simulink model "Rocket_trajectory"  (R2018a)
settings: Solver=ode45  StartTime=0.0  StopTime=360  MinStep=1e-6  RelTol=1e-7
undefined symbols (not defined in the file): Ae, Azimuth, BurnoutInertia, BurnTime, CA, CG, CLL, CLLp, CLNb, CLNr, CMa, CMadot, CMq, CNa, CYb, deg, Earth, Finalcg, Fuel_mass, InertiaRate, InitialInertia, Initialmass, Lat, Launch_angle, Launch_site, Lon, Lref, MACH, Mass_flow, omegajeta, omegalox, rad, Ramup_time, s, Sample_time, Thrust, Thrust_time, Time_cg, Time_slosh, WGS84, Xref
libraries: aerolibconvert2 x6, simulink_extras x5, aerolibbdyn x4, aerolibwind2 x3, aerolibasang x3, aerolibtransform2 x2, aerolibatmos2 x1, shared6dof x1, aerolibfltsims x1, aerolibadyn x1
settings Model: Creator=mario  LastModifiedBy=mario
settings SolverCC: InitialStep=1e-6
settings CodeAppCC: StateflowObjectComments=on

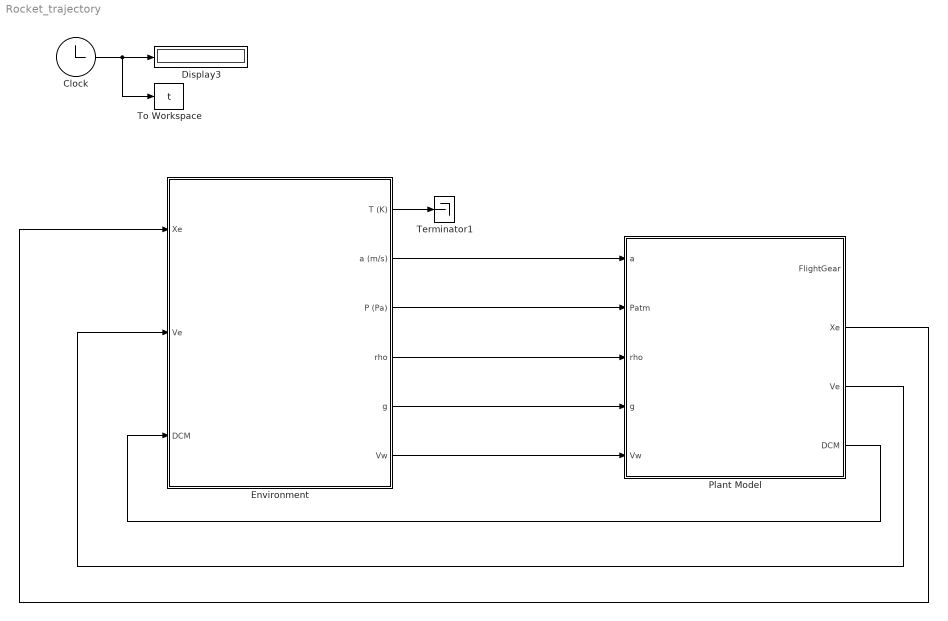
== system Rocket_trajectory ==
  Clock : Clock
  Display3 : Display
  Environment : Subsystem
  Plant Model : Subsystem
  Terminator1 : Terminator
  To Workspace : ToWorkspace  VariableName=t  SampleTime=Sample_time
  wires:
  Environment/3(P (Pa)) -> Plant Model/2(Patm)
  Environment/2(a (m/s)) -> Plant Model/1(a)
  Environment/6(Vw) -> Plant Model/5(Vw)
  Environment/5(g) -> Plant Model/4(g)
  Environment/1(T (K)) -> Terminator1/1
  Clock/1 -> To Workspace/1, Display3/1
  Plant Model/2(Xe) -> Environment/1(Xe)
  Environment/4("rho ") -> Plant Model/3(rho)
  Plant Model/4(DCM) -> Environment/3(DCM)
  Plant Model/3(Ve) -> Environment/2(Ve)

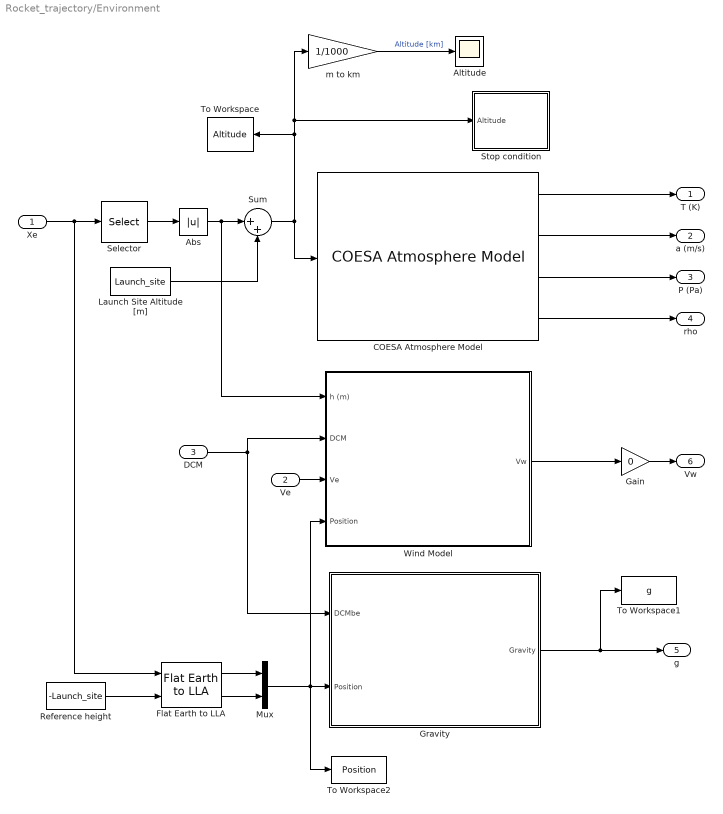
== system Rocket_trajectory/Environment ==
  Xe : Inport
  Ve : Inport  Port=2
  DCM : Inport  Port=3
  Abs : Abs
  Altitude : Scope
  COESA Atmosphere Model : aerolibatmos2/COESA Atmosphere Model  units=Metric (MKS)  spec=1976 COESA-extended U.S. Standard Atmosphere  model=Profile  profile_var=High temperature  profile_percent=1%  profile_alt=5 km (16404 ft)  envelope_var=High temperature  envelope_percent=1%  action=Warning
  Flat Earth to LLA : aerolibtransform2/Flat Earth to LLA  units=Metric (MKS)  ptype=Earth (WGS84)  F=1/298.257223563  R=6378137  LL0=[Lat Lon]  psi=Azimuth
  Gain : Gain  Gain=0
  Gravity : Subsystem
  Launch Site Altitude [m] : Constant  Value=Launch_site
  Mux : Mux  Inputs=2
  Reference height : Constant  Value=-Launch_site
  Selector : Selector  InputPortWidth=3  IndexOptions=Index vector (dialog)  Indices=[3]  OutputSizes=1
  Stop condition : Subsystem
  Sum : Sum  Inputs=|++
  To Workspace : ToWorkspace  VariableName=Altitude  SampleTime=Sample_time
  To Workspace1 : ToWorkspace  VariableName=g  SampleTime=Sample_time
  To Workspace2 : ToWorkspace  VariableName=Position  SampleTime=Sample_time
  Wind Model : Subsystem
  m to km : Gain  Gain=1/1000
  T (K) : Outport
  a (m/s) : Outport  Port=2
  P (Pa) : Outport  Port=3
  "rho " : Outport  Port=4
  g : Outport  Port=5
  Vw : Outport  Port=6
  wires:
  Launch Site Altitude [m]/1 -> Sum/2
  m to km/1 -> Altitude/1  "Altitude [km]"
  Selector/1 -> Abs/1
  COESA Atmosphere Model/2 -> a (m/s)/1
  COESA Atmosphere Model/1 -> T (K)/1
  Abs/1 -> Wind Model/1(h (m)), Sum/1
  Xe/1 -> Selector/1, Flat Earth to LLA/1
  COESA Atmosphere Model/3 -> P (Pa)/1
  COESA Atmosphere Model/4 -> "rho "/1
  Sum/1 -> COESA Atmosphere Model/1, Stop condition/1(Altitude), m to km/1, To Workspace/1
  Ve/1 -> Wind Model/3(Ve)
  Gravity/1(Gravity) -> To Workspace1/1, g/1
  DCM/1 -> Wind Model/2(DCM), Gravity/1(DCMbe)
  Flat Earth to LLA/1 -> Mux/1
  Flat Earth to LLA/2 -> Mux/2
  Mux/1 -> To Workspace2/1, Wind Model/4(Position), Gravity/2(Position)
  Reference height/1 -> Flat Earth to LLA/2
  Gain/1 -> Vw/1
  Wind Model/1(Vw) -> Gain/1

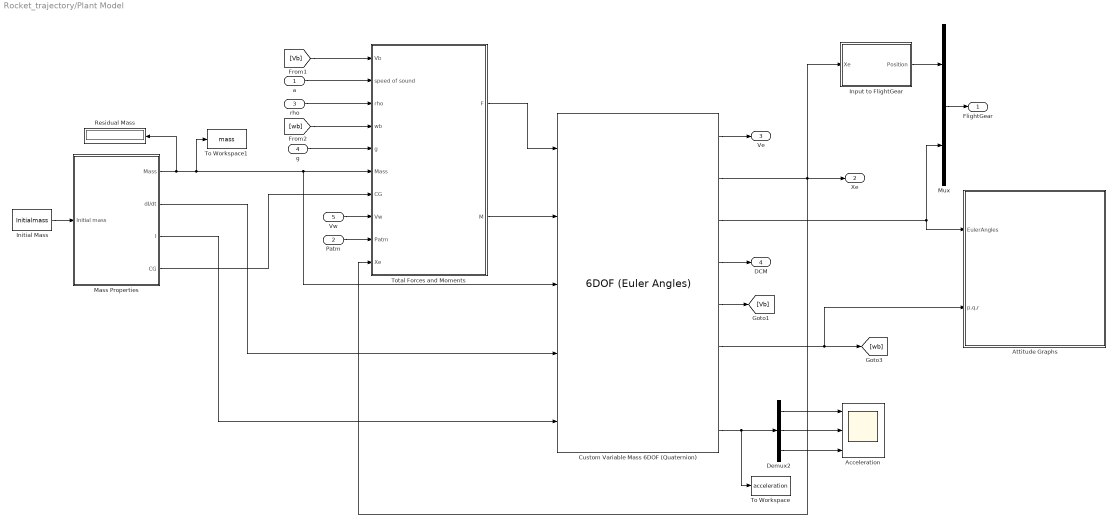
== system Rocket_trajectory/Plant Model ==
  a : Inport
  Patm : Inport  Port=2
  rho : Inport  Port=3
  g : Inport  Port=4
  Vw : Inport  Port=5
  Acceleration : Scope  NumInputPorts=3
  Attitude Graphs : Subsystem
  Custom Variable Mass 6DOF (Quaternion) : shared6dof/6DOF (Euler Angles)  units=Metric (MKS)  mtype=Custom Variable  rep=Quaternion  xme_0=[0 0 0]  Vm_0=[0.1 0.1 0.1]  eul_0=[0 Launch_angle Azimuth]  pm_0=[0 0 0]  mass_0=1.0  mass_e=0.5  mass_f=2.0  inertia=eye(3)  inertia_e=eye(3)  inertia_f=2*eye(3)  k_quat=1.0  vre_flag=off  abi_flag=off  aMode=aMode
      settings: SourceProductBaseCode=AE
  Demux2 : Demux  Outputs=3
  Initial Mass : Constant  Value=Initialmass
  Input to FlightGear : Subsystem
  Mass Properties : Subsystem
  Mux : Mux  Inputs=2
  Residual Mass : Display
  To Workspace : ToWorkspace  VariableName=acceleration  SampleTime=Sample_time
  To Workspace1 : ToWorkspace  VariableName=mass  SampleTime=Sample_time
  "Total Forces and Moments " : Subsystem
  FlightGear : Outport
  Xe : Outport  Port=2
  Ve : Outport  Port=3
  DCM : Outport  Port=4
  wires:
  Custom Variable Mass 6DOF (Quaternion)/4 -> DCM/1
  Mux/1 -> FlightGear/1
  Custom Variable Mass 6DOF (Quaternion)/6 -> [wb], Attitude Graphs/2(p,q,r)
  Custom Variable Mass 6DOF (Quaternion)/1 -> Ve/1
  "Total Forces and Moments "/2("M ") -> Custom Variable Mass 6DOF (Quaternion)/2
  Custom Variable Mass 6DOF (Quaternion)/3 -> Attitude Graphs/1(EulerAngles), Mux/2
  Custom Variable Mass 6DOF (Quaternion)/5 -> [Vb]
  [Vb] -> "Total Forces and Moments "/1("Vb ")
  Input to FlightGear/1(Position) -> Mux/1
  g/1 -> "Total Forces and Moments "/5(g)
  Demux2/3 -> Acceleration/3
  "Total Forces and Moments "/1(F) -> Custom Variable Mass 6DOF (Quaternion)/1
  Custom Variable Mass 6DOF (Quaternion)/2 -> "Total Forces and Moments "/10(Xe), Xe/1, Input to FlightGear/1(Xe)
  [wb] -> "Total Forces and Moments "/4(wb)
  Demux2/2 -> Acceleration/2
  rho/1 -> "Total Forces and Moments "/3("rho ")
  Demux2/1 -> Acceleration/1
  Custom Variable Mass 6DOF (Quaternion)/8 -> To Workspace/1, Demux2/1
  a/1 -> "Total Forces and Moments "/2(speed of sound)
  Mass Properties/2(dI/dt) -> Custom Variable Mass 6DOF (Quaternion)/4
  Initial Mass/1 -> Mass Properties/1(Initial mass)
  Mass Properties/1(Mass) -> To Workspace1/1, Custom Variable Mass 6DOF (Quaternion)/3, "Total Forces and Moments "/6(Mass), Residual Mass/1
  Mass Properties/3(I) -> Custom Variable Mass 6DOF (Quaternion)/5
  Mass Properties/4(CG) -> "Total Forces and Moments "/7(CG)
  Vw/1 -> "Total Forces and Moments "/8(Vw)
  Patm/1 -> "Total Forces and Moments "/9(Patm)

== system Rocket_trajectory/Environment/Gravity ==
  DCMbe : Inport
  Position : Inport  Port=2
  Display4 : Display
  Display5 : Display
  Product3 : Product  Multiplication=Matrix(*)
  "WGS84 Gravity Model  " : GravityWGS84
  Gravity : Outport
  wires:
  Product3/1 -> Gravity/1, Display4/1
  "WGS84 Gravity Model  "/1 -> Product3/2, Display5/1
  DCMbe/1 -> Product3/1
  Position/1 -> "WGS84 Gravity Model  "/1

== system Rocket_trajectory/Environment/Stop condition ==
  Altitude : Inport
  Clock : Clock
  Constant : Constant  Value=0
  Constant1 : Constant
  Constant2 : Constant  Value=Launch_site+10
  Stop Simulation : Stop
  Switch : Switch  Criteria=u2 > Threshold  Threshold=Launch_site+1
  Switch1 : Switch  Criteria=u2 > Threshold  Threshold=10
  wires:
  Switch/1 -> Stop Simulation/1
  Constant/1 -> Switch/1
  Constant1/1 -> Switch/3
  Altitude/1 -> Switch1/1
  Switch1/1 -> Switch/2
  Clock/1 -> Switch1/2
  Constant2/1 -> Switch1/3

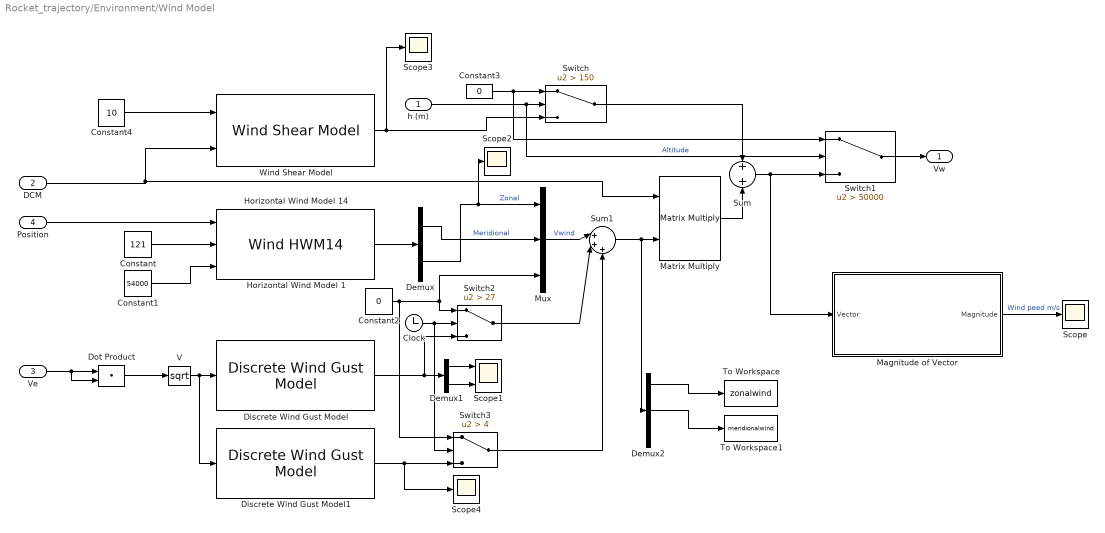
== system Rocket_trajectory/Environment/Wind Model ==
  h (m) : Inport
  DCM : Inport  Port=2
  Ve : Inport  Port=3
  Position : Inport  Port=4
  Clock : Clock
  Constant : Constant  Value=121
  Constant1 : Constant  Value=54000
  Constant2 : Constant  Value=0
  Constant3 : Constant  Value=0
  Constant4 : Constant  Value=10
  Demux : Demux  Outputs=2
  Demux1 : Demux  Outputs=2
  Demux2 : Demux  Outputs=3
  Discrete Wind Gust Model : aerolibwind2/Discrete Wind Gust Model  units=Metric (MKS)  Gx=on  Gy=on  Gz=off  t_0=20  d_m=[150 150 50]  v_m=[10 0 0]
      settings: SourceProductName=Aerospace Blockset
  Discrete Wind Gust Model1 : aerolibwind2/Discrete Wind Gust Model  units=Metric (MKS)  Gx=on  Gy=on  Gz=off  t_0=1  d_m=[20 20 8]  v_m=[10 0 0]
      settings: SourceProductName=Aerospace Blockset
  Dot Product : DotProduct  SaturateOnIntegerOverflow=on  OutDataTypeStr=Inherit: Inherit via internal rule
  Horizontal Wind Model 1 : WindHWM14
  Horizontal Wind Model 14 : WindHWM14
  Magnitude of Vector : Subsystem
  Matrix Multiply : Product  Multiplication=Matrix(*)
  Mux : Mux  Inputs=3
  Scope{,2..4} (4 alike) : Scope
  Scope1 : Scope  NumInputPorts=2
  Sum : Sum
  Sum1 : Sum  Inputs=|+++
  Switch : Switch  Criteria=u2 > Threshold  Threshold=150
  Switch1 : Switch  Criteria=u2 > Threshold  Threshold=50000
  Switch2 : Switch  Criteria=u2 > Threshold  Threshold=27
  Switch3 : Switch  Criteria=u2 > Threshold  Threshold=4
  To Workspace : ToWorkspace  VariableName=zonalwind  SampleTime=Sample_time
  To Workspace1 : ToWorkspace  VariableName=meridionalwind  SampleTime=Sample_time
  V : Math  Operator=sqrt  SaturateOnIntegerOverflow=on
  Wind Shear Model : aerolibwind2/Wind Shear Model  units=Metric (MKS)  phase=Category C - Terminal Flight Phase  W_20=10  Wdeg=20
      settings: SourceProductName=Aerospace Blockset
  Vw : Outport
  wires:
  Ve/1 -> Dot Product/2, Dot Product/1
  Dot Product/1 -> V/1
  Magnitude of Vector/1(Magnitude) -> Scope/1  "Wind peed m/s"
  Discrete Wind Gust Model/1 -> Switch2/3, Demux1/1
  Position/1 -> Horizontal Wind Model 14/1
  Constant/1 -> Horizontal Wind Model 14/2
  Constant1/1 -> Horizontal Wind Model 14/3
  Horizontal Wind Model 14/1 -> Demux/1
  Demux/1 -> Mux/2  "Meridional"
  Demux/2 -> Scope2/1, Mux/1  "Zonal"
  Demux1/1 -> Scope1/1
  Demux1/2 -> Scope1/2
  DCM/1 -> Wind Shear Model/2, Matrix Multiply/1
  Mux/1 -> Sum1/1  "Vwind"
  Matrix Multiply/1 -> Sum/2
  h (m)/1 -> Switch1/2, Switch/2  "Altitude"
  Sum/1 -> Switch1/3, Magnitude of Vector/1(Vector)
  Wind Shear Model/1 -> Scope3/1, Switch/3
  Switch/1 -> Sum/1
  Constant3/1 -> Switch1/1, Switch/1
  Constant4/1 -> Wind Shear Model/1
  Switch1/1 -> Vw/1
  Sum1/1 -> Demux2/1, Matrix Multiply/2
  Switch2/1 -> Sum1/2
  Demux2/1 -> To Workspace/1
  Demux2/2 -> To Workspace1/1
  V/1 -> Discrete Wind Gust Model1/1, Discrete Wind Gust Model/1
  Discrete Wind Gust Model1/1 -> Scope4/1, Switch3/3
  Clock/1 -> Switch3/2, Switch2/2
  Constant2/1 -> Switch3/1, Mux/3, Switch2/1
  Switch3/1 -> Sum1/3

== system Rocket_trajectory/Plant Model/Attitude Graphs ==
  EulerAngles : Inport
  p,q,r : Inport  Port=2
  Angular Rates : Scope  NumInputPorts=3
  Atittude : Scope  NumInputPorts=6
  Demux : Demux  Outputs=3
  Demux1 : Demux  Outputs=3
  Euler Angles : Scope  NumInputPorts=3
  "Roll, Pitch, Yaw" : simulink_extras/Transformations/Radians to Degrees
  wires:
  Demux/1 -> Atittude/1, Euler Angles/1  "Roll"
  "Roll, Pitch, Yaw"/1 -> Demux/1
  Demux1/3 -> Angular Rates/3, Atittude/6  "Yaw rate"
  Demux1/2 -> Angular Rates/2, Atittude/5  "Pitch rate"
  Demux/3 -> Atittude/3, Euler Angles/3  "Yaw"
  Demux/2 -> Atittude/2, Euler Angles/2  "Pitch"
  Demux1/1 -> Angular Rates/1, Atittude/4  "Roll rate"
  EulerAngles/1 -> "Roll, Pitch, Yaw"/1
  p,q,r/1 -> Demux1/1

== system Rocket_trajectory/Plant Model/Input to FlightGear ==
  Xe : Inport
  Constant2 : Constant  Value=-Launch_site
  Demux2 : Demux  Outputs=2
  Demux3 : Demux  Outputs=3
  Flat Earth to LLA : aerolibtransform2/Flat Earth to LLA  units=Metric (MKS)  ptype=Earth (WGS84)  F=1/298.257223563  R=6378137  LL0=[Lat Lon]  psi=0
  Generate Run Script : aerolibfltsims/Generate Run Script  Architecture=Win64  dataFlow=Send  GeometryModelName=sr71  AirportId=KSFO  RunwayId=10L  InitialAltitude=4593  InitialHeading=0  OffsetDistance=4.72  OffsetAzimuth=0  InstallScenery=off  DisableShaders=off  OriginAddress=127.0.0.1  DestinationPort=5502  OriginPort=5505  LocalAddress=127.0.0.1  OutputFileName=runfg.bat  FlightGearBaseDirectory=C:\Program Files\FlightGear 2017.3.1
  Mux1 : Mux  Inputs=3
  Mux2 : Mux  Inputs=3
  Position : Outport
  wires:
  Demux3/3 -> Mux1/3
  Demux3/1 -> Mux1/1
  Flat Earth to LLA/2 -> Mux2/3
  Xe/1 -> Demux3/1
  Demux2/1 -> Mux2/2
  Demux2/2 -> Mux2/1
  Flat Earth to LLA/1 -> Demux2/1
  Constant2/1 -> Flat Earth to LLA/2
  Mux1/1 -> Flat Earth to LLA/1
  Demux3/2 -> Mux1/2
  Mux2/1 -> Position/1

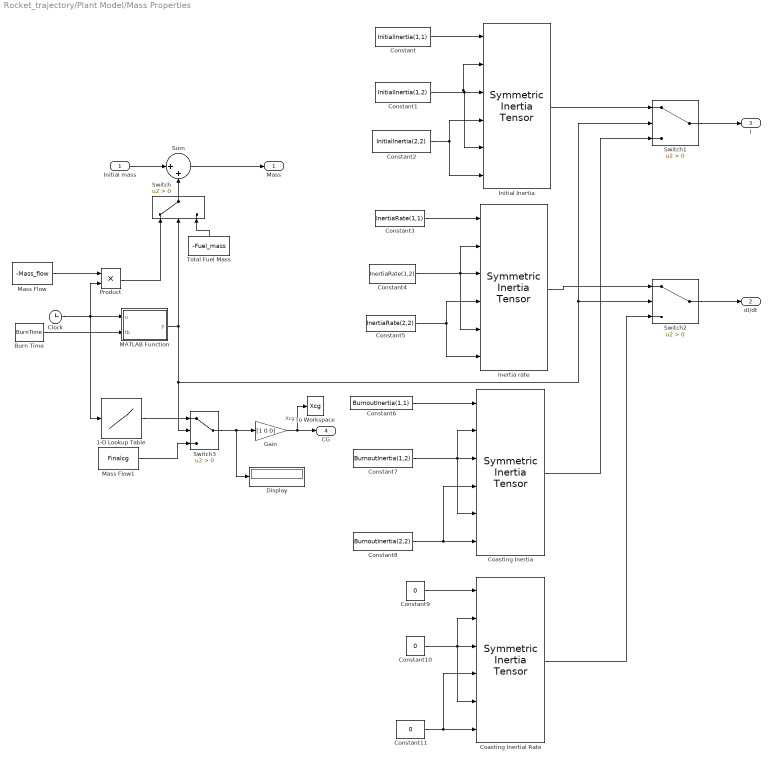
== system Rocket_trajectory/Plant Model/Mass Properties ==
  Initial mass : Inport
  1-D Lookup Table : Lookup_n-D  NumberOfTableDimensions=1  BreakpointsForDimension1=Time_cg  Table=CG  InternalRulePriority=Speed  RndMeth=Simplest  InputSameDT=on
  Burn Time : Constant  Value=BurnTime
  Clock : Clock
  Coasting Inertia : aerolibbdyn/Symmetric Inertia Tensor
      settings: SourceProductName=Aerospace Blockset  SourceProductBaseCode=AE
  Coasting Inertial Rate : aerolibbdyn/Symmetric Inertia Tensor
      settings: SourceProductName=Aerospace Blockset  SourceProductBaseCode=AE
  Constant : Constant  Value=InitialInertia(1,1)
  Constant1 : Constant  Value=InitialInertia(1,2)
  Constant10 : Constant  Value=0
  Constant11 : Constant  Value=0
  Constant2 : Constant  Value=InitialInertia(2,2)
  Constant3 : Constant  Value=InertiaRate(1,1)
  Constant4 : Constant  Value=InertiaRate(1,2)
  Constant5 : Constant  Value=InertiaRate(2,2)
  Constant6 : Constant  Value=BurnoutInertia(1,1)
  Constant7 : Constant  Value=BurnoutInertia(1,2)
  Constant8 : Constant  Value=BurnoutInertia(2,2)
  Constant9 : Constant  Value=0
  Display : Display
  Gain : Gain  Gain=[1 0 0]
  Inertia rate : aerolibbdyn/Symmetric Inertia Tensor
      settings: SourceProductName=Aerospace Blockset  SourceProductBaseCode=AE
  Initial Inertia : aerolibbdyn/Symmetric Inertia Tensor
      settings: SourceProductName=Aerospace Blockset  SourceProductBaseCode=AE
  MATLAB Function : MATLAB Function  TreatAsAtomicUnit=on
  Mass Flow : Constant  Value=-Mass_flow
  Mass Flow1 : Constant  Value=Finalcg
  Product : Product
  Sum : Sum  Inputs=|++
  Switch{,1..3} (4 alike) : Switch  Criteria=u2 > Threshold
  To Workspace : ToWorkspace  VariableName=Xcg  SampleTime=Sample_time
  Total Fuel Mass : Constant  Value=-Fuel_mass
  Mass : Outport
  dI/dt : Outport  Port=2
  I : Outport  Port=3
  CG : Outport  Port=4
  wires:
  Initial mass/1 -> Sum/1
  Constant/1 -> Initial Inertia/1
  Constant1/1 -> Initial Inertia/5, Initial Inertia/2, Initial Inertia/3
  Constant2/1 -> Initial Inertia/4, Initial Inertia/6
  Mass Flow/1 -> Product/1
  Clock/1 -> 1-D Lookup Table/1, Product/2, MATLAB Function/1(u)
  Product/1 -> Switch/1
  Constant5/1 -> Inertia rate/4, Inertia rate/6
  Constant3/1 -> Inertia rate/1
  Constant4/1 -> Inertia rate/2, Inertia rate/5, Inertia rate/3
  Inertia rate/1 -> Switch2/1
  Sum/1 -> Mass/1
  Switch/1 -> Sum/2
  Total Fuel Mass/1 -> Switch/3
  Burn Time/1 -> MATLAB Function/2(tb)
  Coasting Inertia/1 -> Switch1/3
  Constant8/1 -> Coasting Inertia/4, Coasting Inertia/6
  Constant6/1 -> Coasting Inertia/1
  Constant7/1 -> Coasting Inertia/5, Coasting Inertia/2, Coasting Inertia/3
  Initial Inertia/1 -> Switch1/1
  Switch1/1 -> I/1
  Switch2/1 -> dI/dt/1
  Constant11/1 -> Coasting Inertial Rate/4, Coasting Inertial Rate/6
  Constant9/1 -> Coasting Inertial Rate/1
  Constant10/1 -> Coasting Inertial Rate/2, Coasting Inertial Rate/3, Coasting Inertial Rate/5
  Coasting Inertial Rate/1 -> Switch2/3
  1-D Lookup Table/1 -> Switch3/1
  Switch3/1 -> Gain/1, Display/1
  MATLAB Function/1(y) -> Switch3/2, Switch2/2, Switch1/2, Switch/2
  Mass Flow1/1 -> Switch3/3
  Gain/1 -> To Workspace/1, CG/1  "Xcg"

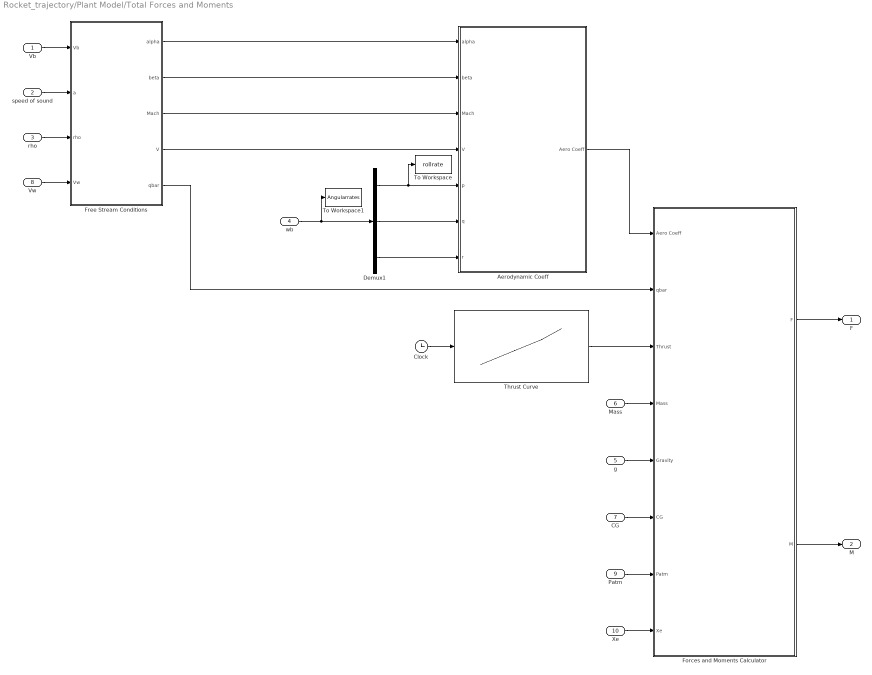
== system Rocket_trajectory/Plant Model/Total Forces and Moments  ==
  "Vb " : Inport
  speed of sound : Inport  Port=2
  "rho " : Inport  Port=3
  wb : Inport  Port=4
  g : Inport  Port=5
  Mass : Inport  Port=6
  CG : Inport  Port=7
  Vw : Inport  Port=8
  Patm : Inport  Port=9
  Xe : Inport  Port=10
  Aerodynamic Coeff : Subsystem
  Clock : Clock
  Demux1 : Demux  Outputs=3
  Forces and Moments Calculator : Subsystem
  Free Stream Conditions : Subsystem
  "Thrust Curve " : Lookup_n-D  NumberOfTableDimensions=1  BreakpointsForDimension1=Thrust_time  Table=Thrust  InternalRulePriority=Speed  RndMeth=Simplest  InputSameDT=on
  To Workspace : ToWorkspace  VariableName=rollrate  SampleTime=Sample_time
  To Workspace1 : ToWorkspace  VariableName=Angularrates  SampleTime=-1
  F : Outport
  "M " : Outport  Port=2
  wires:
  Aerodynamic Coeff/1(Aero Coeff) -> Forces and Moments Calculator/1(Aero Coeff)
  Forces and Moments Calculator/1(F) -> F/1
  Forces and Moments Calculator/2(M) -> "M "/1
  Mass/1 -> Forces and Moments Calculator/4(Mass)
  "Thrust Curve "/1 -> Forces and Moments Calculator/3(Thrust)
  Clock/1 -> "Thrust Curve "/1
  Demux1/3 -> Aerodynamic Coeff/7(r)
  Demux1/2 -> Aerodynamic Coeff/6(q)
  wb/1 -> To Workspace1/1, Demux1/1
  Demux1/1 -> To Workspace/1, Aerodynamic Coeff/5(p)
  g/1 -> Forces and Moments Calculator/5(Gravity)
  "Vb "/1 -> Free Stream Conditions/1(Vb)
  speed of sound/1 -> Free Stream Conditions/2(a)
  "rho "/1 -> Free Stream Conditions/3(rho)
  Free Stream Conditions/1(alpha) -> Aerodynamic Coeff/1(alpha)
  Free Stream Conditions/2(beta) -> Aerodynamic Coeff/2(beta)
  Free Stream Conditions/3(Mach) -> Aerodynamic Coeff/3(Mach)
  Free Stream Conditions/4(V) -> Aerodynamic Coeff/4(V)
  Free Stream Conditions/5(qbar) -> Forces and Moments Calculator/2(qbar)
  CG/1 -> Forces and Moments Calculator/6(CG)
  Vw/1 -> Free Stream Conditions/4(Vw)
  Patm/1 -> Forces and Moments Calculator/7(Patm)
  Xe/1 -> Forces and Moments Calculator/8(Xe)

== system Rocket_trajectory/Environment/Wind Model/Magnitude of Vector ==
  Vector : Inport
  Demux : Demux  Outputs=3
  Multiply : Product
  Multiply1 : Product
  Multiply2 : Product
  Sqrt : Sqrt  SaturateOnIntegerOverflow=on
  Sum1 : Sum  Inputs=3
  Magnitude : Outport
  wires:
  Demux/1 -> Multiply/2, Multiply/1
  Sum1/1 -> Sqrt/1
  Demux/2 -> Multiply1/1, Multiply1/2
  Multiply1/1 -> Sum1/2
  Sqrt/1 -> Magnitude/1
  Demux/3 -> Multiply2/2, Multiply2/1
  Multiply2/1 -> Sum1/3
  Multiply/1 -> Sum1/1
  Vector/1 -> Demux/1

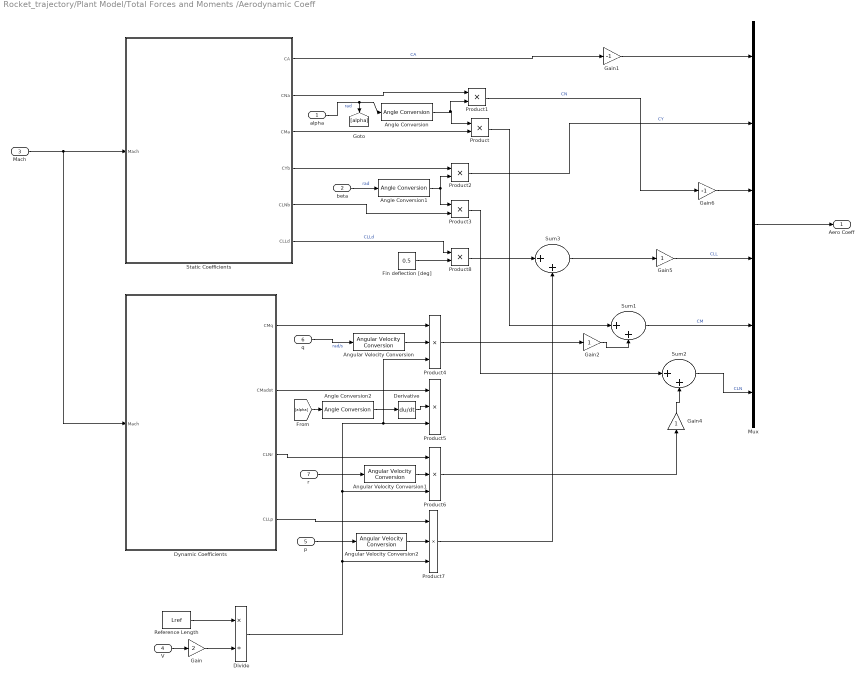
== system Rocket_trajectory/Plant Model/Total Forces and Moments /Aerodynamic Coeff ==
  alpha : Inport
  beta : Inport  Port=2
  Mach : Inport  Port=3
  V : Inport  Port=4
  p : Inport  Port=5
  q : Inport  Port=6
  r : Inport  Port=7
  Angle Conversion : aerolibconvert2/Angle Conversion  IU=rad  OU=deg
  Angle Conversion1 : aerolibconvert2/Angle Conversion  IU=rad  OU=deg
  Angle Conversion2 : aerolibconvert2/Angle Conversion  IU=rad  OU=deg
  Angular Velocity Conversion : aerolibconvert2/Angular Velocity Conversion  IU=rad/s  OU=deg/s
      settings: SourceProductName=Aerospace Blockset
  Angular Velocity Conversion1 : aerolibconvert2/Angular Velocity Conversion  IU=rad/s  OU=deg/s
      settings: SourceProductName=Aerospace Blockset
  Angular Velocity Conversion2 : aerolibconvert2/Angular Velocity Conversion  IU=rad/s  OU=deg/s
      settings: SourceProductName=Aerospace Blockset
  Derivative : Derivative
  Divide : Product  Inputs=*/
  Dynamic Coefficients : Subsystem
  Fin deflection [deg] : Constant  Value=0.5
  Gain : Gain  Gain=2
  Gain1 : Gain  Gain=-1
  Gain2 : Gain
  Gain4 : Gain
  Gain5 : Gain
  Gain6 : Gain  Gain=-1
  Mux : Mux  Inputs=6
  Product{,1..3,8} (5 alike) : Product
  Product{4..7} (4 alike) : Product  Inputs=3
  Reference Length : Constant  Value=Lref
  "Static Coefficients " : Subsystem
  Sum1 : Sum  Inputs=|++
  Sum2 : Sum  Inputs=|++
  Sum3 : Sum  Inputs=|++
  Aero Coeff : Outport
  wires:
  Mach/1 -> "Static Coefficients "/1(Mach), Dynamic Coefficients/1(Mach)
  Dynamic Coefficients/1("CMq ") -> Product4/1
  Mux/1 -> Aero Coeff/1
  "Static Coefficients "/1("CA ") -> Gain1/1  "CA"
  Product1/1 -> Gain6/1  "CN"
  "Static Coefficients "/6("CLLd  ") -> Product8/1  "CLLd"
  Sum1/1 -> Mux/5  "CM"
  Sum2/1 -> Mux/6  "CLN"
  alpha/1 -> Angle Conversion/1, [alpha]  "rad"
  "Static Coefficients "/3("CMa ") -> Product/2
  "Static Coefficients "/2("CNa ") -> Product1/1
  beta/1 -> Angle Conversion1/1  "rad"
  "Static Coefficients "/5("CLNb ") -> Product3/2
  "Static Coefficients "/4("CYb ") -> Product2/1
  Product2/1 -> Mux/2  "CY"
  Product/1 -> Sum1/1
  Reference Length/1 -> Divide/1
  V/1 -> Gain/1
  Gain/1 -> Divide/2
  [alpha] -> Angle Conversion2/1
  Divide/1 -> Product7/3, Product6/3, Product4/3, Product5/3
  Product4/1 -> Gain2/1
  Dynamic Coefficients/2("CMadot ") -> Product5/1
  q/1 -> Angular Velocity Conversion/1  "rad/s"
  Dynamic Coefficients/3("CLNr ") -> Product6/1
  r/1 -> Angular Velocity Conversion1/1
  Derivative/1 -> Product5/2
  Product6/1 -> Gain4/1
  Product3/1 -> Sum2/1
  Gain1/1 -> Mux/1
  Angle Conversion/1 -> Product/1, Product1/2
  Angle Conversion1/1 -> Product3/1, Product2/2
  Angle Conversion2/1 -> Derivative/1
  Angular Velocity Conversion/1 -> Product4/2
  Angular Velocity Conversion1/1 -> Product6/2
  Gain2/1 -> Sum1/2
  Gain4/1 -> Sum2/2
  Gain5/1 -> Mux/4  "CLL"
  Gain6/1 -> Mux/3
  Sum3/1 -> Gain5/1
  Dynamic Coefficients/4(CLLp) -> Product7/1
  Angular Velocity Conversion2/1 -> Product7/2
  p/1 -> Angular Velocity Conversion2/1
  Product7/1 -> Sum3/2
  Product8/1 -> Sum3/1
  Fin deflection [deg]/1 -> Product8/2

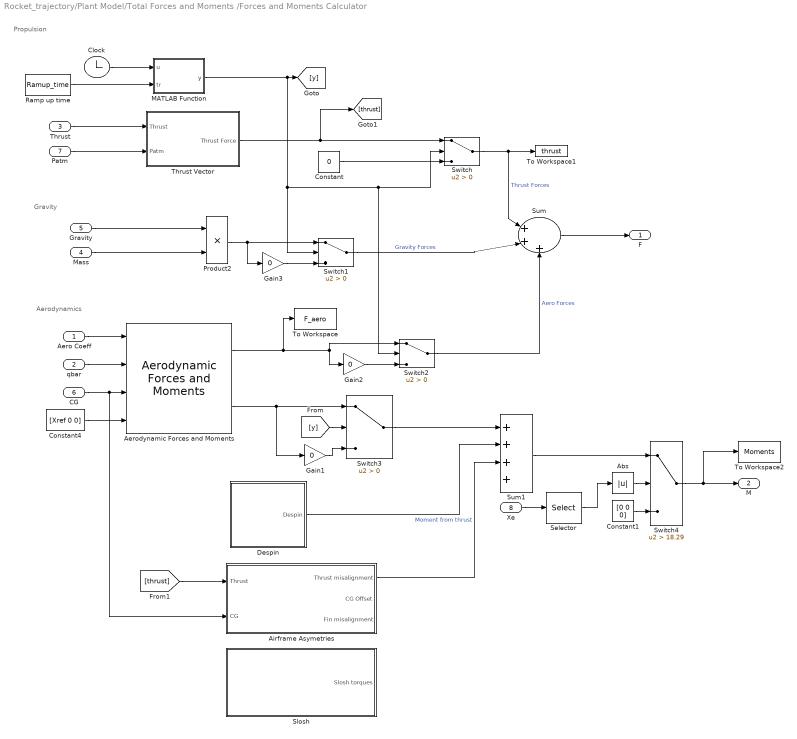
== system Rocket_trajectory/Plant Model/Total Forces and Moments /Forces and Moments Calculator ==
  note: Propulsion
  note: Gravity
  note: Aerodynamics
  Aero Coeff : Inport
  qbar : Inport  Port=2
  Thrust : Inport  Port=3
  Mass : Inport  Port=4
  Gravity : Inport  Port=5
  CG : Inport  Port=6
  Patm : Inport  Port=7
  Xe : Inport  Port=8
  Abs : Abs
  "Aerodynamic Forces and Moments " : aerolibadyn/Aerodynamic Forces and Moments   inputAxes=Body  outputForceAxes=Body  outputMomentAxes=Body  S=Aref  b=Lref  cbar=Lref
      settings: SourceProductName=Aerospace Blockset
  Airframe Asymetries : Subsystem
  Clock : Clock
  Constant : Constant  Value=0
  Constant1 : Constant  Value=[0 0 0]
  Constant4 : Constant  Value=[Xref 0 0]
  Despin : Subsystem
  Gain1 : Gain  Gain=0
  Gain2 : Gain  Gain=0
  Gain3 : Gain  Gain=0
  MATLAB Function : MATLAB Function  TreatAsAtomicUnit=on
  Product2 : Product
  Ramp up time : Constant  Value=Ramup_time
  Selector : Selector  InputPortWidth=3  IndexOptions=Index vector (dialog)  Indices=[3]  OutputSizes=1
  Slosh : Subsystem
  Sum : Sum  Inputs=|+++
  Sum1 : Sum  Inputs=++++
  Switch{,1..3} (4 alike) : Switch  Criteria=u2 > Threshold
  Switch4 : Switch  Criteria=u2 > Threshold  Threshold=18.29
  Thrust Vector : Subsystem
  To Workspace : ToWorkspace  VariableName=F_aero  SampleTime=Sample_time
  To Workspace1 : ToWorkspace  VariableName=thrust  SampleTime=Sample_time
      settings: Save2DSignal=2-D array (concatenate along first dimension)
  To Workspace2 : ToWorkspace  VariableName=Moments  SampleTime=Sample_time
  F : Outport
  M : Outport  Port=2
  wires:
  Aero Coeff/1 -> "Aerodynamic Forces and Moments "/1
  Thrust/1 -> Thrust Vector/1(Thrust)
  Sum/1 -> F/1
  Gravity/1 -> Product2/1
  Mass/1 -> Product2/2
  Product2/1 -> Gain3/1, Switch1/1
  Constant/1 -> Switch/3
  Clock/1 -> MATLAB Function/1(u)
  Ramp up time/1 -> MATLAB Function/2(tr)
  MATLAB Function/1(y) -> [y], Switch/2, Switch2/2, Switch1/2
  Switch/1 -> To Workspace1/1, Sum/1  "Thrust Forces"
  Switch3/1 -> Sum1/1
  Gain1/1 -> Switch3/3
  Gain2/1 -> Switch2/3
  Switch2/1 -> Sum/3  "Aero Forces"
  Gain3/1 -> Switch1/3
  Switch1/1 -> Sum/2  "Gravity Forces"
  [y] -> Switch3/2
  Sum1/1 -> Switch4/1
  "Aerodynamic Forces and Moments "/1 -> To Workspace/1, Switch2/1, Gain2/1
  "Aerodynamic Forces and Moments "/2 -> Gain1/1, Switch3/1
  Constant4/1 -> "Aerodynamic Forces and Moments "/4
  CG/1 -> Airframe Asymetries/2(CG), "Aerodynamic Forces and Moments "/3
  qbar/1 -> "Aerodynamic Forces and Moments "/2
  Despin/1("Despin ") -> Sum1/2
  [thrust] -> Airframe Asymetries/1(Thrust)
  Airframe Asymetries/1("Thrust misalignment ") -> Sum1/3  "Moment from thrust"
  Thrust Vector/1("Thrust Force ") -> [thrust], Switch/1
  Patm/1 -> Thrust Vector/2(Patm)
  Selector/1 -> Abs/1
  Xe/1 -> Selector/1
  Abs/1 -> Switch4/2
  Switch4/1 -> To Workspace2/1, M/1
  Constant1/1 -> Switch4/3

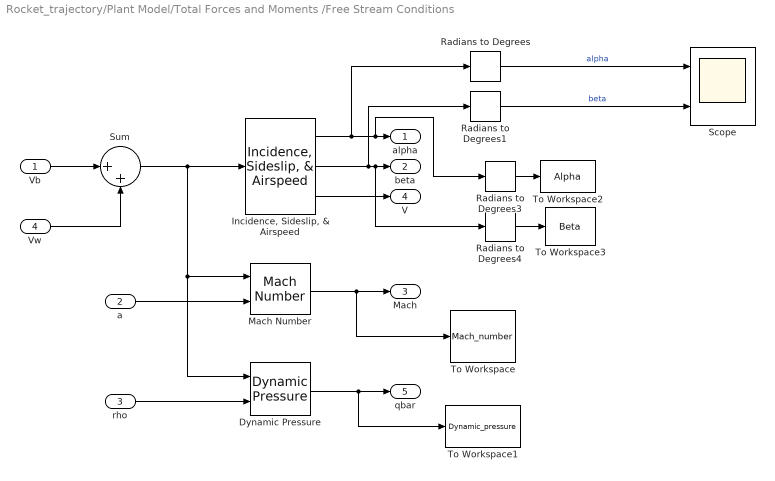
== system Rocket_trajectory/Plant Model/Total Forces and Moments /Free Stream Conditions ==
  Vb : Inport
  a : Inport  Port=2
  rho : Inport  Port=3
  Vw : Inport  Port=4
  Dynamic Pressure : aerolibasang/Dynamic Pressure
  "Incidence, Sideslip, & Airspeed" : aerolibasang/Incidence, Sideslip, & Airspeed
      settings: SourceProductName=Aerospace Blockset
  Mach Number : aerolibasang/Mach Number
      settings: SourceProductName=Aerospace Blockset  SourceProductBaseCode=AE
  Radians to Degrees{,1,3..4} (4 alike) : simulink_extras/Transformations/Radians to Degrees
  Scope : Scope  NumInputPorts=2
  Sum : Sum  Inputs=|++
  To Workspace : ToWorkspace  VariableName=Mach_number  SampleTime=Sample_time
  To Workspace1 : ToWorkspace  VariableName=Dynamic_pressure  SampleTime=Sample_time
  To Workspace2 : ToWorkspace  VariableName=Alpha  SampleTime=-1
  To Workspace3 : ToWorkspace  VariableName=Beta  SampleTime=-1
  alpha : Outport
  beta : Outport  Port=2
  Mach : Outport  Port=3
  V : Outport  Port=4
  qbar : Outport  Port=5
  wires:
  Mach Number/1 -> To Workspace/1, Mach/1
  Sum/1 -> Dynamic Pressure/1, Mach Number/1, "Incidence, Sideslip, & Airspeed"/1
  "Incidence, Sideslip, & Airspeed"/1 -> Radians to Degrees/1, Radians to Degrees3/1, alpha/1
  Vb/1 -> Sum/1
  Dynamic Pressure/1 -> To Workspace1/1, qbar/1
  "Incidence, Sideslip, & Airspeed"/3 -> V/1
  a/1 -> Mach Number/2
  "Incidence, Sideslip, & Airspeed"/2 -> Radians to Degrees1/1, Radians to Degrees4/1, beta/1
  rho/1 -> Dynamic Pressure/2
  Radians to Degrees/1 -> Scope/1  "alpha"
  Vw/1 -> Sum/2
  Radians to Degrees1/1 -> Scope/2  "beta"
  Radians to Degrees3/1 -> To Workspace2/1
  Radians to Degrees4/1 -> To Workspace3/1

== system Rocket_trajectory/Plant Model/Total Forces and Moments /Aerodynamic Coeff/Dynamic Coefficients ==
  Mach : Inport
  "CLLp " : Lookup_n-D  NumberOfTableDimensions=1  BreakpointsForDimension1=MACH  Table=CLLp  InternalRulePriority=Speed  RndMeth=Simplest  InputSameDT=on
  CLNr : Lookup_n-D  NumberOfTableDimensions=1  BreakpointsForDimension1=MACH  Table=CLNr  InternalRulePriority=Speed  RndMeth=Simplest  InputSameDT=on
  CMadot : Lookup_n-D  NumberOfTableDimensions=1  BreakpointsForDimension1=MACH  Table=CMadot  InternalRulePriority=Speed  RndMeth=Simplest  InputSameDT=on
  CMq+CMadot : Lookup_n-D  NumberOfTableDimensions=1  BreakpointsForDimension1=MACH  Table=CMq  InternalRulePriority=Speed  RndMeth=Simplest  InputSameDT=on
  "CMq " : Outport
  "CMadot " : Outport  Port=2
  "CLNr " : Outport  Port=3
  CLLp : Outport  Port=4
  wires:
  Mach/1 -> "CLLp "/1, CLNr/1, CMadot/1, CMq+CMadot/1
  CMadot/1 -> "CMadot "/1
  CMq+CMadot/1 -> "CMq "/1
  CLNr/1 -> "CLNr "/1
  "CLLp "/1 -> CLLp/1

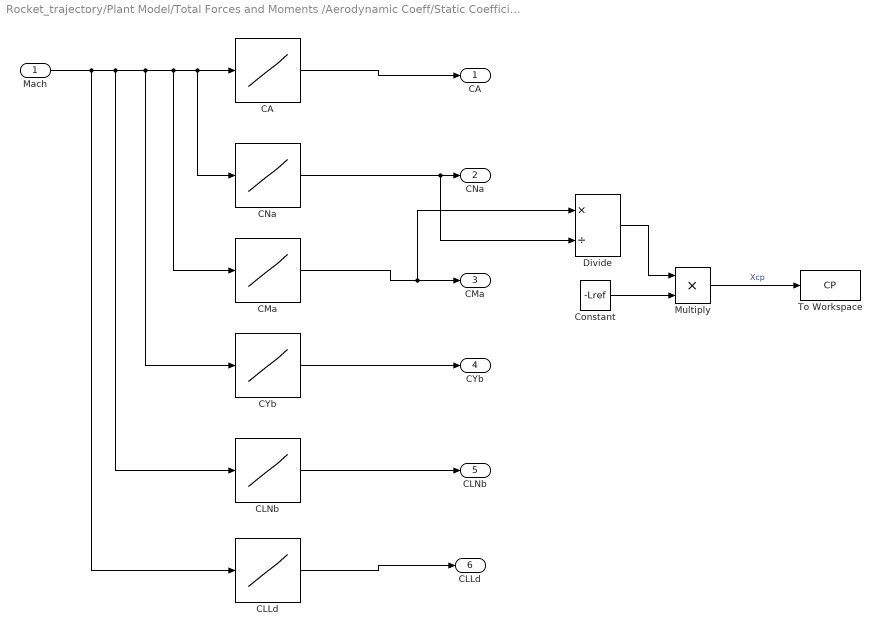
== system Rocket_trajectory/Plant Model/Total Forces and Moments /Aerodynamic Coeff/Static Coefficients  ==
  Mach : Inport
  CA : Lookup_n-D  NumberOfTableDimensions=1  BreakpointsForDimension1=MACH  Table=CA  InternalRulePriority=Speed  RndMeth=Simplest  InputSameDT=on
  CLLd : Lookup_n-D  NumberOfTableDimensions=1  BreakpointsForDimension1=MACH  Table=CLL  InternalRulePriority=Speed  RndMeth=Simplest  InputSameDT=on
  CLNb : Lookup_n-D  NumberOfTableDimensions=1  BreakpointsForDimension1=MACH  Table=CLNb  InternalRulePriority=Speed  RndMeth=Simplest  InputSameDT=on
  CMa : Lookup_n-D  NumberOfTableDimensions=1  BreakpointsForDimension1=MACH  Table=CMa  InternalRulePriority=Speed  RndMeth=Simplest  InputSameDT=on
  CNa : Lookup_n-D  NumberOfTableDimensions=1  BreakpointsForDimension1=MACH  Table=CNa  InternalRulePriority=Speed  RndMeth=Simplest  InputSameDT=on
  CYb : Lookup_n-D  NumberOfTableDimensions=1  BreakpointsForDimension1=MACH  Table=CYb  InternalRulePriority=Speed  RndMeth=Simplest  InputSameDT=on
  Constant : Constant  Value=-Lref
  Divide : Product  Inputs=*/
  Multiply : Product
  To Workspace : ToWorkspace  VariableName=CP  SampleTime=Sample_time
  "CA " : Outport
  "CNa " : Outport  Port=2
  "CMa " : Outport  Port=3
  "CYb " : Outport  Port=4
  "CLNb " : Outport  Port=5
  "CLLd  " : Outport  Port=6
  wires:
  Mach/1 -> CLLd/1, CLNb/1, CYb/1, CMa/1, CNa/1, CA/1
  CA/1 -> "CA "/1
  CNa/1 -> Divide/2, "CNa "/1
  CMa/1 -> Divide/1, "CMa "/1
  CYb/1 -> "CYb "/1
  CLNb/1 -> "CLNb "/1
  CLLd/1 -> "CLLd  "/1
  Multiply/1 -> To Workspace/1  "Xcp"
  Divide/1 -> Multiply/1
  Constant/1 -> Multiply/2

== system Rocket_trajectory/Plant Model/Total Forces and Moments /Forces and Moments Calculator/Airframe Asymetries ==
  Thrust : Inport
  CG : Inport  Port=2
  CG Misalignment : Subsystem
  Gain1 : Gain  Gain=0
  Gain2 : Gain  Gain=0
  Gain3 : Gain  Gain=0
  Subsystem : Subsystem
  Sum : Sum  Inputs=++|
  Thrust Misalignment : Subsystem
  "Thrust misalignment " : Outport
  CG Offset : Outport  Port=2
  Fin misalignment : Outport  Port=3
  wires:
  Sum/1 -> "Thrust misalignment "/1
  Gain1/1 -> Sum/2
  Gain2/1 -> Sum/1
  Gain3/1 -> CG Offset/1
  CG/1 -> Thrust Misalignment/2(CG)
  Thrust Misalignment/1(Offset) -> Gain2/1
  Thrust Misalignment/2(Angle) -> Gain1/1
  Subsystem/1(Moment_CGoffset) -> Gain3/1
  Thrust/1 -> Thrust Misalignment/1(Thrust), Subsystem/1(Thrust)

== system Rocket_trajectory/Plant Model/Total Forces and Moments /Forces and Moments Calculator/Despin ==
  Clock1 : Clock
  Constant1 : Constant  Value=59
  Constant3 : Constant  Value=0
  Despin : Constant  Value=-210
  Gain4 : Gain  Gain=[1 0 0]
  MATLAB Function1 : MATLAB Function  TreatAsAtomicUnit=on
  Switch4 : Switch  Criteria=u2 > Threshold
  "Despin " : Outport
  wires:
  Constant1/1 -> MATLAB Function1/2(td)
  Constant3/1 -> Switch4/1
  Despin/1 -> Switch4/3
  Gain4/1 -> "Despin "/1
  MATLAB Function1/1(y) -> Switch4/2
  Clock1/1 -> MATLAB Function1/1(u)
  Switch4/1 -> Gain4/1

== system Rocket_trajectory/Plant Model/Total Forces and Moments /Forces and Moments Calculator/Slosh ==
  1-D Lookup Table : Lookup_n-D  NumberOfTableDimensions=1  BreakpointsForDimension1=Time_slosh  Table=omegajeta  InternalRulePriority=Speed  RndMeth=Simplest  InputSameDT=on
  1-D Lookup Table1 : Lookup_n-D  NumberOfTableDimensions=1  BreakpointsForDimension1=Time_slosh  Table=omegalox  InternalRulePriority=Speed  RndMeth=Simplest  InputSameDT=on
  Clock : Clock
  Constant : Constant  Value=0
  Scope : Scope  NumInputPorts=2
  Switch : Switch  Criteria=u2 > Threshold  Threshold=27
  Switch1 : Switch  Criteria=u2 > Threshold  Threshold=27
  Slosh torques : Outport
  wires:
  Clock/1 -> Switch/2, Switch1/2, 1-D Lookup Table1/1, 1-D Lookup Table/1
  1-D Lookup Table/1 -> Switch/3  "Jet A natural frequency"
  1-D Lookup Table1/1 -> Switch1/3  "LOX natural frequency"
  Constant/1 -> Switch1/1, Switch/1
  Switch/1 -> Scope/1
  Switch1/1 -> Scope/2

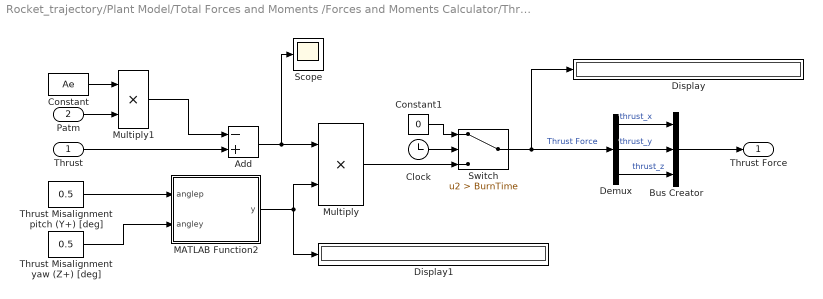
== system Rocket_trajectory/Plant Model/Total Forces and Moments /Forces and Moments Calculator/Thrust Vector ==
  Thrust : Inport
  Patm : Inport  Port=2
  Add : Sum  Inputs=-+
  Bus Creator : BusCreator  Inputs=3
  Clock : Clock
  Constant : Constant  Value=Ae
  Constant1 : Constant  Value=0
  Demux : Demux  Outputs=3
  Display : Display
  Display1 : Display
  MATLAB Function2 : MATLAB Function  TreatAsAtomicUnit=on
  Multiply : Product
  Multiply1 : Product
  Scope : Scope
  Switch : Switch  Criteria=u2 > Threshold  Threshold=BurnTime
  Thrust Misalignment pitch (Y+) [deg] : Constant  Value=0.5
  Thrust Misalignment yaw (Z+) [deg] : Constant  Value=0.5
  "Thrust Force " : Outport
  wires:
  Thrust/1 -> Add/2
  Multiply/1 -> Switch/3
  Thrust Misalignment pitch (Y+) [deg]/1 -> MATLAB Function2/1(anglep)
  MATLAB Function2/1(y) -> Display1/1, Multiply/2
  Thrust Misalignment yaw (Z+) [deg]/1 -> MATLAB Function2/2(angley)
  Add/1 -> Scope/1, Multiply/1
  Patm/1 -> Multiply1/2
  Constant/1 -> Multiply1/1
  Multiply1/1 -> Add/1
  Clock/1 -> Switch/2
  Constant1/1 -> Switch/1
  Switch/1 -> Display/1, Demux/1  "Thrust Force"
  Bus Creator/1 -> "Thrust Force "/1
  Demux/1 -> Bus Creator/1  "thrust_x"
  Demux/2 -> Bus Creator/2  "thrust_y"
  Demux/3 -> Bus Creator/3  "thrust_z"

== system Rocket_trajectory/Plant Model/Total Forces and Moments /Forces and Moments Calculator/Airframe Asymetries/CG Misalignment ==
  note: CG offset must be entered positive if its position is in the Z+ or Y+ axis in the body frame coordinate
  In Bus Element : Inport  PortName=Thrust  Element=thrust_x
  In Bus Element1 : Inport  PortName=Thrust  Element=thrust_y
  In Bus Element2 : Inport  PortName=Thrust  Element=thrust_z
  CG offset in Y : Constant  Value=0.01
  CG offset in Z : Constant  Value=0.01
  Gain : Gain  Gain=-1
  Multiply{,1..3} (4 alike) : Product
  Mux2 : Mux  Inputs=3
  Sum : Sum  Inputs=++|
  Moment_CGoffset : Outport
  wires:
  Multiply2/1 -> Sum/1
  Multiply3/1 -> Sum/2
  Sum/1 -> Mux2/1
  Multiply1/1 -> Mux2/3
  Gain/1 -> Mux2/2
  In Bus Element2/1 -> Multiply3/1
  In Bus Element1/1 -> Multiply2/1
  In Bus Element/1 -> Multiply/1, Multiply1/1
  CG offset in Y/1 -> Multiply1/2, Multiply3/2
  CG offset in Z/1 -> Multiply/2, Multiply2/2
  Multiply/1 -> Gain/1
  Mux2/1 -> Moment_CGoffset/1

== system Rocket_trajectory/Plant Model/Total Forces and Moments /Forces and Moments Calculator/Airframe Asymetries/Subsystem ==
  note: CG offset must be entered positive if its position is in the Z+ or Y+ axis in the body frame coordinate
  In Bus Element : Inport  PortName=Thrust  Element=thrust_x
  In Bus Element1 : Inport  PortName=Thrust  Element=thrust_y
  In Bus Element2 : Inport  PortName=Thrust  Element=thrust_z
  CG offset in Y : Constant  Value=0.01
  CG offset in Z : Constant  Value=0.01
  Gain : Gain  Gain=-1
  Gain1 : Gain  Gain=-1
  Multiply{,1..3} (4 alike) : Product
  Mux2 : Mux  Inputs=3
  Sum : Sum  Inputs=++|
  Moment_CGoffset : Outport
  wires:
  Mux2/1 -> Moment_CGoffset/1
  Multiply/1 -> Gain/1
  CG offset in Z/1 -> Multiply2/2, Multiply/2
  Multiply1/1 -> Gain1/1
  CG offset in Y/1 -> Multiply3/2, Multiply1/2
  In Bus Element/1 -> Multiply1/1, Multiply/1
  In Bus Element1/1 -> Multiply2/1
  In Bus Element2/1 -> Multiply3/1
  Gain/1 -> Mux2/2
  Gain1/1 -> Mux2/3
  Sum/1 -> Mux2/1
  Multiply3/1 -> Sum/2
  Multiply2/1 -> Sum/1

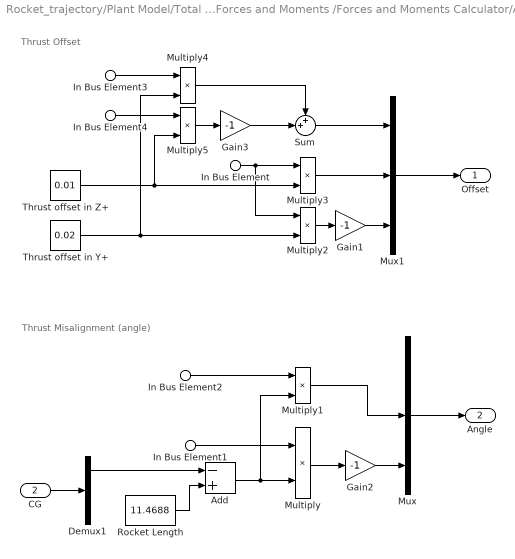
== system Rocket_trajectory/Plant Model/Total Forces and Moments /Forces and Moments Calculator/Airframe Asymetries/Thrust Misalignment ==
  note: Thrust Offset
  note: Thrust Misalignment (angle)
  In Bus Element : Inport  PortName=Thrust  Element=thrust_x
  In Bus Element1 : Inport  PortName=Thrust  Element=thrust_y
  In Bus Element4 : Inport  PortName=Thrust  Element=thrust_y
  In Bus Element2 : Inport  PortName=Thrust  Element=thrust_z
  In Bus Element3 : Inport  PortName=Thrust  Element=thrust_z
  CG : Inport  Port=2
  Add : Sum  Inputs=-+
  Demux1 : Demux  Outputs=3
  Gain1 : Gain  Gain=-1
  Gain2 : Gain  Gain=-1
  Gain3 : Gain  Gain=-1
  Multiply{,1..5} (6 alike) : Product
  Mux : Mux  Inputs=3
  Mux1 : Mux  Inputs=3
  Rocket Length : Constant  Value=11.4688
  Sum : Sum  Inputs=++|
  Thrust offset in Y+ : Constant  Value=0.02
  Thrust offset in Z+ : Constant  Value=0.01
  Offset : Outport
  Angle : Outport  Port=2
  wires:
  In Bus Element/1 -> Multiply2/1, Multiply3/1
  Mux1/1 -> Offset/1
  Mux/1 -> Angle/1
  Multiply3/1 -> Mux1/2
  Demux1/1 -> Add/1
  Add/1 -> Multiply1/2, Multiply/2
  CG/1 -> Demux1/1
  Multiply1/1 -> Mux/2
  Multiply/1 -> Gain2/1
  Rocket Length/1 -> Add/2
  In Bus Element1/1 -> Multiply/1
  Thrust offset in Z+/1 -> Multiply5/2, Multiply3/2
  In Bus Element2/1 -> Multiply1/1
  Thrust offset in Y+/1 -> Multiply4/2, Multiply2/2
  Gain1/1 -> Mux1/3
  Multiply2/1 -> Gain1/1
  Gain2/1 -> Mux/3
  In Bus Element3/1 -> Multiply4/1
  In Bus Element4/1 -> Multiply5/1
  Sum/1 -> Mux1/1
  Multiply5/1 -> Gain3/1
  Multiply4/1 -> Sum/1
  Gain3/1 -> Sum/2

== matlab function Rocket_trajectory/Plant Model/Total Forces and Moments /Forces and Moments Calculator/Thrust Vector/MATLAB Function2 ==
  data: anglep input; y output; angley input
function y = fcn(anglep, angley)

axial= cos(deg2rad(anglep))*cos(deg2rad(angley));

pitch =sin(deg2rad(anglep));

yaw = sin(deg2rad(angley));
y=[axial,yaw,pitch];

end

== matlab function Rocket_trajectory/Plant Model/Total Forces and Moments /Forces and Moments Calculator/MATLAB Function ==
  data: u input; y output; tr input
function y = fcn(u, tr)
if u<=tr
    y=0;
else 
    y=1;

end

== matlab function Rocket_trajectory/Plant Model/Mass Properties/MATLAB Function ==
  data: u input; y output; tb input
function y = fcn(u,tb)
if u>=tb
    
    y=0;
    
else
    y=1;

end

== matlab function Rocket_trajectory/Plant Model/Total Forces and Moments /Forces and Moments Calculator/Despin/MATLAB Function1 ==
  data: u input; y output; td input
function y = fcn(u, td)
if u>=td && u<=60
    y=0;
else 
    y=1;

end
